simulink library "AEMS_Standard_Library"  (R2016b)
settings: Solver=ode45  StartTime=0.0  StopTime=10.0  RelTol=1e-3
undefined symbols (not defined in the file or in its folder): BkPY, carto, Cbx_extegr, Cbx_lpegrsys, Cbx_portegr, Cnx_bnk_nr_conf, Cnx_cyl_nr_conf, ConfigManagement, configuration_management, Cxx_dcm_io_tmr_end_xxxx, Cxx_dcm_rt_tmr_end, Cxx_DID_xxxx_IO_max, Cxx_DID_xxxx_IO_min, Cxx_egrhsofs, Cxx_vmaniegi, DEM_DEBOUNCE_FREEZE, DEM_DTR_CTL_INVISIBLE, DEM_DTR_CTL_NORMAL, Dem_DtrId2_XXX, Dem_DtrId3_XXX, Dem_DtrId4_XXX, Dem_DtrId5_XXX, Dem_DtrId6_XXX, Dem_DtrId7_XXX, Dem_DtrId8_XXX, Dem_DtrId9_XXX, Dem_DtrId_XXX, Dem_EnableConditionId2_XXX, Dem_EnableConditionId3_XXX, Dem_EnableConditionId4_XXX, Dem_EnableConditionId5_XXX, Dem_EnableConditionId6_XXX, Dem_EnableConditionId7_XXX, Dem_EnableConditionId8_XXX, Dem_EnableConditionId_XXX, Dem_EventId, Dem_EventId2_XXX, Dem_EventId3_XXX, Dem_EventId4_XXX, Dem_EventId5_XXX, Dem_EventId6_XXX, Dem_EventId7_XXX, Dem_EventId8_XXX, Dem_EventId9_XXX, Dem_EventId_Device_Faulttype, Dem_EventId_XXX, DEM_IUMPR_GENERAL_DENOMINATOR, DEM_OPCYC_IGNITION, Dem_RatioId2_XXX, Dem_RatioId3_XXX, Dem_RatioId4_XXX, Dem_RatioId5_XXX, Dem_RatioId6_XXX, Dem_RatioId7_XXX, Dem_RatioId8_XXX, Dem_RatioId_XXX, Dem_StorageConditionId2_XXX, Dem_StorageConditionId3_XXX, Dem_StorageConditionId4_XXX, Dem_StorageConditionId5_XXX ... (+65)
libraries: AEMS_Standard_Library x477, simulink x2
(part 19 of 39)

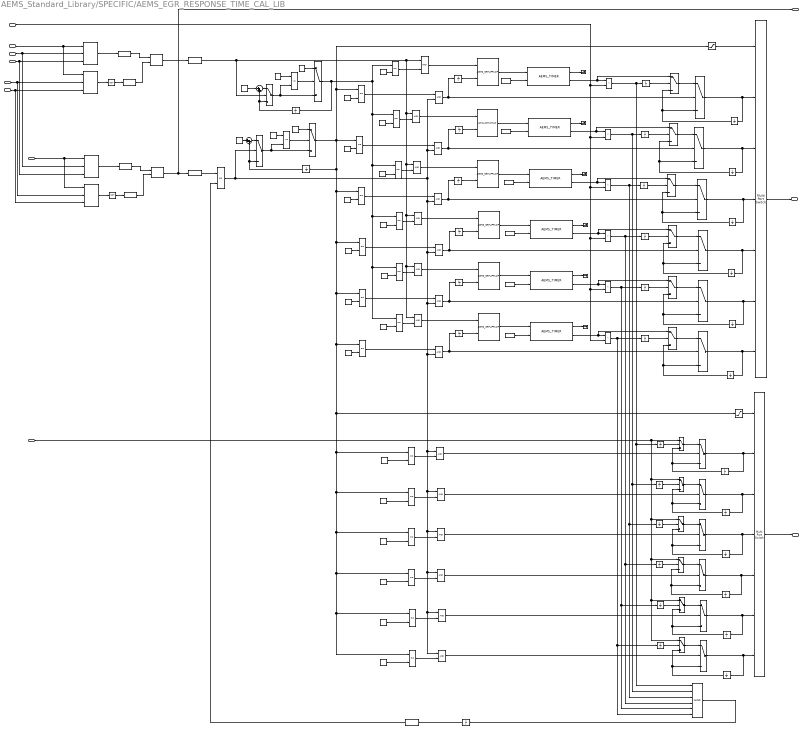
== system AEMS_Standard_Library/SPECIFIC/AEMS_EGR_RESPONSE_TIME_CAL_LIB ==
  timeup_time : Inport  PortDimensions=1
      settings: AttributesFormatString=<tsample=%<SampleTime>>
  etdamsf : Inport  Port=2  PortDimensions=1
      settings: AttributesFormatString=<tsample=%<SampleTime>>
  goal_trig_parameter : Inport  Port=3  PortDimensions=1
      settings: AttributesFormatString=<tsample=%<SampleTime>>
  start_trig_parameter : Inport  Port=4  PortDimensions=1
      settings: AttributesFormatString=<tsample=%<SampleTime>>
  on_thrs : Inport  Port=5  PortDimensions=1
      settings: AttributesFormatString=<tsample=%<SampleTime>>
  off_thrs : Inport  Port=6  PortDimensions=1
      settings: AttributesFormatString=<tsample=%<SampleTime>>
  on_hysw : Inport  Port=7  PortDimensions=1
      settings: AttributesFormatString=<tsample=%<SampleTime>>
  off_hysw : Inport  Port=8  PortDimensions=1
      settings: AttributesFormatString=<tsample=%<SampleTime>>
  AEMS_EDGE_EITHER1 : AEMS_Standard_Library/EDGE/AEMS_EDGE_EITHER  Tag=[LIB]  init=false
      settings: AttributesFormatString=|
      | %<MaskType>
      | Initial Value : %<init>
  AEMS_EDGE_EITHER2 : AEMS_Standard_Library/EDGE/AEMS_EDGE_EITHER  Tag=[LIB]  init=false
      settings: AttributesFormatString=|
      | %<MaskType>
      | Initial Value : %<init>
  AEMS_EDGE_RISING{,1..4} (5 alike) : AEMS_Standard_Library/EDGE/AEMS_EDGE_RISING  Tag=[LIB]  init=false
      settings: AttributesFormatString=|
      | %<MaskType>
      | Initial Value : %<init>
  AEMS_HYST_DELTARIGHT1 : AEMS_Standard_Library/HYSTERESIS/AEMS_HYST_DELTARIGHT  Tag=[LIB]
      settings: AttributesFormatString=%<MaskType>
  AEMS_HYST_DELTARIGHT2 : AEMS_Standard_Library/HYSTERESIS/AEMS_HYST_DELTARIGHT  Tag=[LIB]
      settings: AttributesFormatString=%<MaskType>
  AEMS_HYST_LEFTDELTA1 : AEMS_Standard_Library/HYSTERESIS/AEMS_HYST_LEFTDELTA  Tag=[LIB]
      settings: AttributesFormatString=%<MaskType>
  AEMS_HYST_LEFTDELTA2 : AEMS_Standard_Library/HYSTERESIS/AEMS_HYST_LEFTDELTA  Tag=[LIB]
      settings: AttributesFormatString=%<MaskType>
  AEMS_SRFLIPFLOP{,1..7} (8 alike) : AEMS_Standard_Library/FLAG/AEMS_SRFLIPFLOP  Tag=[LIB]  init=false
      settings: AttributesFormatString=%<MaskType>\nInitial condition (state of Q): = %<init>
  AEMS_TIMER{,1..5} (6 alike) : AEMS_Standard_Library/TIMER/AEMS_TIMER  Tag=[LIB]  sample_time=0.01
      settings: AttributesFormatString=%<MaskType>
  Constant10 : Constant  Value=6  OutDataTypeStr=uint8
  Constant11 : Constant  Value=6  OutDataTypeStr=uint8
  Constant12 : Constant  Value=4  OutDataTypeStr=uint8
  Constant13 : Constant  Value=5  OutDataTypeStr=uint8
  Constant14 : Constant  Value=6  OutDataTypeStr=uint8
  Constant{3,6,9,16..18} (6 alike) : Constant  OutDataTypeStr=single
  Constant{19,21..22,25,29,32..33} (7 alike) : Constant  OutDataTypeStr=uint8
  Constant20 : Constant  Value=7  OutDataTypeStr=uint8
  Constant23 : Constant  Value=2  OutDataTypeStr=uint8
  Constant24 : Constant  Value=3  OutDataTypeStr=uint8
  Constant26 : Constant  Value=2  OutDataTypeStr=uint8
  Constant27 : Constant  Value=3  OutDataTypeStr=uint8
  Constant28 : Constant  Value=7  OutDataTypeStr=uint8
  Constant30 : Constant  Value=3  OutDataTypeStr=uint8
  Constant31 : Constant  Value=2  OutDataTypeStr=uint8
  Constant4 : Constant  Value=4  OutDataTypeStr=uint8
  Constant5 : Constant  Value=4  OutDataTypeStr=uint8
  Constant7 : Constant  Value=5  OutDataTypeStr=uint8
  Constant8 : Constant  Value=5  OutDataTypeStr=uint8
  Logical Operator{1,4..11,13,17,19,24..29} (18 alike) : Logic  OutDataTypeStr=boolean
  Logical Operator12 : Logic  Operator=NOT  OutDataTypeStr=boolean
  Logical Operator18 : Logic  Operator=NAND  Inputs=6  OutDataTypeStr=boolean
  Logical Operator2 : Logic  Operator=OR  OutDataTypeStr=boolean
  Logical Operator3 : Logic  Operator=NOT  OutDataTypeStr=boolean
  Multiport Switch : MultiPortSwitch  Inputs=6  SaturateOnIntegerOverflow=on  InputSameDT=on
  Multiport Switch1 : MultiPortSwitch  Inputs=6  SaturateOnIntegerOverflow=on  InputSameDT=on
  Relational Operator{2,5..6,8,10..14,20,22..23,25..26,28..31} (18 alike) : RelationalOperator  Operator===  OutDataTypeStr=boolean  RndMeth=Nearest  InputSameDT=on
  Relational Operator{16,18..19,21,24,27} (6 alike) : RelationalOperator  Operator=<  OutDataTypeStr=boolean  RndMeth=Nearest  InputSameDT=on
  Relational Operator7 : RelationalOperator  Operator=<=  OutDataTypeStr=boolean  RndMeth=Nearest  InputSameDT=on
  Relational Operator9 : RelationalOperator  Operator=<=  OutDataTypeStr=boolean  RndMeth=Nearest  InputSameDT=on
  Saturation : Saturate  UpperLimit=6  LowerLimit=1
      settings: AttributesFormatString=<limits=%<UpperLimit>/%<LowerLimit>>
  Saturation1 : Saturate  UpperLimit=6  LowerLimit=1
      settings: AttributesFormatString=<limits=%<UpperLimit>/%<LowerLimit>>
  Sum1 : Sum  Inputs=|++  SaturateOnIntegerOverflow=on
  Sum2 : Sum  Inputs=|++  SaturateOnIntegerOverflow=on
  Switch{,1..10,12..13,15..17,20..31} (28 alike) : Switch  Threshold=0.5  SaturateOnIntegerOverflow=on  InputSameDT=on
      Switch settings: AttributesFormatString=<Threshold=%<Threshold>>
      Switch1 settings: AttributesFormatString=<threshold=%<threshold>>
      Switch10 settings: AttributesFormatString=<threshold=%<threshold>>
      Switch12 settings: AttributesFormatString=<threshold=%<threshold>>
      Switch13 settings: AttributesFormatString=<threshold=%<threshold>>
      Switch15 settings: AttributesFormatString=<Threshold=%<Threshold>>
      Switch16 settings: AttributesFormatString=<Threshold=%<Threshold>>
      Switch17 settings: AttributesFormatString=<Threshold=%<Threshold>>
      Switch2 settings: AttributesFormatString=<Threshold=%<Threshold>>
      Switch20 settings: AttributesFormatString=<Threshold=%<Threshold>>
      Switch21 settings: AttributesFormatString=<Threshold=%<Threshold>>
      Switch22 settings: AttributesFormatString=<Threshold=%<Threshold>>
      Switch23 settings: AttributesFormatString=<Threshold=%<Threshold>>
      Switch24 settings: AttributesFormatString=<Threshold=%<Threshold>>
      Switch25 settings: AttributesFormatString=<Threshold=%<Threshold>>
      Switch26 settings: AttributesFormatString=<threshold=%<threshold>>
      Switch27 settings: AttributesFormatString=<threshold=%<threshold>>
      Switch28 settings: AttributesFormatString=<threshold=%<threshold>>
      Switch29 settings: AttributesFormatString=<threshold=%<threshold>>
      Switch3 settings: AttributesFormatString=<Threshold=%<Threshold>>
      Switch30 settings: AttributesFormatString=<threshold=%<threshold>>
      Switch31 settings: AttributesFormatString=<threshold=%<threshold>>
      Switch4 settings: AttributesFormatString=<threshold=%<threshold>>
      Switch5 settings: AttributesFormatString=<threshold=%<threshold>>
      Switch6 settings: AttributesFormatString=<threshold=%<threshold>>
      Switch7 settings: AttributesFormatString=<threshold=%<threshold>>
      Switch8 settings: AttributesFormatString=<threshold=%<threshold>>
      Switch9 settings: AttributesFormatString=<threshold=%<threshold>>
  Terminator{,1..5} (6 alike) : Terminator
  Unit Delay{,1,3,7..14,16..23,25..38} (33 alike) : UnitDelay  SampleTime=-1
      settings: AttributesFormatString=<initial=%<X0>>
  fegrqinc : Outport  PortDimensions=1
  egrqpassdt : Outport  Port=2  PortDimensions=1
  etdamsf_store : Outport  Port=3  PortDimensions=1
  wires:
  Unit Delay14/1 -> Sum1/2, Switch12/3  "count_pudt"
  Unit Delay1/1 -> Sum2/2, Switch1/3  "count1_pudt"
  AEMS_SRFLIPFLOP6/1 -> fegrqinc/1, AEMS_EDGE_EITHER2/1  "fegrqinc"
  AEMS_EDGE_RISING4/1 -> AEMS_SRFLIPFLOP6/2
  AEMS_EDGE_RISING3/1 -> AEMS_SRFLIPFLOP6/1
  Logical Operator12/1 -> AEMS_EDGE_RISING4/1  "flag"
  AEMS_HYST_LEFTDELTA2/1 -> Logical Operator12/1  "egrq0_off"
  AEMS_HYST_DELTARIGHT2/1 -> AEMS_EDGE_RISING3/1  "egrq0_on"
  goal_trig_parameter/1 -> AEMS_HYST_LEFTDELTA2/1, AEMS_HYST_DELTARIGHT2/1  "goal_trig_parameter"
  off_thrs/1 -> AEMS_HYST_LEFTDELTA2/2, AEMS_HYST_LEFTDELTA1/2  "off_thrs"
  AEMS_EDGE_RISING2/1 -> AEMS_SRFLIPFLOP3/2
  AEMS_EDGE_RISING/1 -> AEMS_SRFLIPFLOP3/1
  Logical Operator3/1 -> AEMS_EDGE_RISING2/1  "flag"
  AEMS_HYST_LEFTDELTA1/1 -> Logical Operator3/1  "egrq0_off"
  off_hysw/1 -> AEMS_HYST_LEFTDELTA2/3, AEMS_HYST_LEFTDELTA1/3  "off_hysw"
  AEMS_HYST_DELTARIGHT1/1 -> AEMS_EDGE_RISING/1  "egrq0_on"
  on_hysw/1 -> AEMS_HYST_DELTARIGHT2/3, AEMS_HYST_DELTARIGHT1/3  "on_hysw"
  on_thrs/1 -> AEMS_HYST_DELTARIGHT2/2, AEMS_HYST_DELTARIGHT1/2  "on_thrs"
  start_trig_parameter/1 -> AEMS_HYST_DELTARIGHT1/1, AEMS_HYST_LEFTDELTA1/1  "start_trig_parameter"
  AEMS_EDGE_RISING1/1 -> Logical Operator2/2
  Switch/1 -> Unit Delay/1, Multiport Switch1/2  "holdtime1"
  AEMS_TIMER/1 -> Terminator/1
  Constant18/1 -> AEMS_TIMER/2  "target_time"
  Switch12/1 -> Relational Operator9/2, Switch13/3  "add"
  Constant20/1 -> Relational Operator9/1
  Constant21/1 -> Switch13/1
  Relational Operator9/1 -> Switch13/2
  Switch13/1 -> Relational Operator10/1, Relational Operator11/1, Relational Operator20/1, Relational Operator23/1, Relational Operator26/1, Relational Operator14/1, Unit Delay14/1  "count"
  Relational Operator14/1 -> Logical Operator4/2
  Constant22/1 -> Relational Operator14/2
  Constant23/1 -> Relational Operator10/2
  Relational Operator10/1 -> Logical Operator6/2
  Constant24/1 -> Relational Operator11/2
  Relational Operator11/1 -> Logical Operator7/2
  Constant19/1 -> Sum1/1
  Sum1/1 -> Switch12/1
  Switch2/1 -> Multiport Switch1/3, Unit Delay7/1  "holdtime2"
  AEMS_TIMER1/1 -> Terminator1/1
  Constant16/1 -> AEMS_TIMER1/2  "target_time"
  Switch3/1 -> Unit Delay8/1, Multiport Switch1/4  "holdtime3"
  AEMS_TIMER2/1 -> Terminator2/1
  Constant17/1 -> AEMS_TIMER2/2  "target_time"
  Unit Delay9/1 -> Switch9/3, Switch4/3  "hold2_z"
  Switch4/1 -> Unit Delay9/1, Multiport Switch/3  "hold2"
  Constant26/1 -> Relational Operator2/2
  Unit Delay11/1 -> Switch10/3, Switch6/3  "hold3_z"
  Switch6/1 -> Unit Delay11/1, Multiport Switch/4  "hold3"
  Constant27/1 -> Relational Operator6/2
  Switch5/1 -> Unit Delay10/1, Multiport Switch/2  "hold1"
  Unit Delay10/1 -> Switch5/3, Switch8/3  "hod1_z"
  Saturation/1 -> Multiport Switch/1
  Constant25/1 -> Relational Operator5/2
  Saturation1/1 -> Multiport Switch1/1
  Multiport Switch/1 -> etdamsf_store/1  "etdamsf_store"
  AEMS_SRFLIPFLOP/1 -> AEMS_TIMER/1  "start_flag"
  Logical Operator4/1 -> AEMS_SRFLIPFLOP/1  "set"
  Logical Operator8/1 -> Unit Delay13/1, Switch/2  "fhold1"
  AEMS_SRFLIPFLOP1/1 -> AEMS_TIMER1/1  "start_flag"
  Logical Operator6/1 -> AEMS_SRFLIPFLOP1/1  "set"
  AEMS_SRFLIPFLOP2/1 -> AEMS_TIMER2/1  "start_flag"
  Logical Operator7/1 -> AEMS_SRFLIPFLOP2/1  "set"
  Logical Operator5/1 -> Unit Delay12/1, Switch2/2  "fhold2"
  Logical Operator1/1 -> Unit Delay3/1, Switch3/2  "fhold3"
  Switch1/1 -> Switch7/3, Relational Operator7/2  "add1"
  Constant28/1 -> Relational Operator7/1
  Constant29/1 -> Switch7/1
  Relational Operator7/1 -> Switch7/2
  Sum2/1 -> Switch1/1
  Constant30/1 -> Relational Operator8/2
  Constant31/1 -> Relational Operator12/2
  Constant32/1 -> Relational Operator13/2
  Relational Operator8/1 -> Logical Operator1/1  "store_clear3"
  Relational Operator13/1 -> Logical Operator8/1  "store_clear1"
  Relational Operator12/1 -> Logical Operator5/1  "store_clear2"
  Relational Operator5/1 -> Logical Operator9/2
  Logical Operator9/1 -> Switch5/2
  Relational Operator2/1 -> Logical Operator10/2
  Logical Operator10/1 -> Switch4/2
  Relational Operator6/1 -> Logical Operator11/2
  Logical Operator11/1 -> Switch6/2
  Unit Delay3/1 -> AEMS_SRFLIPFLOP2/2  "clear"
  Unit Delay12/1 -> AEMS_SRFLIPFLOP1/2  "clear"
  Unit Delay13/1 -> AEMS_SRFLIPFLOP/2  "clear"
  Unit Delay/1 -> Switch/3, Switch16/3  "holdtime1_z"
  Unit Delay8/1 -> Switch3/3, Switch17/3  "holdtime3_z"
  Multiport Switch1/1 -> egrqpassdt/1  "egrqpassdt"
  AEMS_TIMER1/2 -> Relational Operator16/1, Switch15/1
  Relational Operator16/1 -> Unit Delay17/1, Unit Delay22/1, Logical Operator18/2  "timeok2"
  Unit Delay7/1 -> Switch15/3, Switch2/3  "holdtime2_z"
  Switch15/1 -> Switch2/1
  Constant33/1 -> Sum2/1
  Logical Operator18/1 -> Unit Delay18/1  "ftimeover"
  Logical Operator2/1 -> Switch1/2, Logical Operator8/2, Logical Operator5/2, Logical Operator1/2, Logical Operator13/2, Logical Operator19/2, Logical Operator25/2, Logical Operator9/1, Logical Operator11/1, Logical Operator27/1, Logical Operator28/1, Logical Operator29/1, Logical Operator10/1  "time_stop"
  Unit Delay18/1 -> AEMS_EDGE_RISING1/1  "flag"
  Relational Operator18/1 -> Unit Delay23/1, Logical Operator18/3, Unit Delay20/1  "timeok3"
  Switch17/1 -> Switch3/1
  AEMS_TIMER2/2 -> Relational Operator18/1, Switch17/1
  AEMS_TIMER/2 -> Switch16/1, Relational Operator19/1
  Switch16/1 -> Switch/1
  Relational Operator19/1 -> Unit Delay21/1, Logical Operator18/1, Unit Delay19/1  "timeok1"
  timeup_time/1 -> Relational Operator16/2, Relational Operator18/2, Relational Operator21/2, Relational Operator24/2, Relational Operator27/2, Relational Operator19/2  "timeup_time"
  Switch8/1 -> Switch5/1
  Switch9/1 -> Switch4/1
  Switch10/1 -> Switch6/1
  etdamsf/1 -> Switch8/1, Switch9/1, Switch10/1, Switch26/1, Switch28/1, Switch30/1  "etdamsf"
  AEMS_SRFLIPFLOP3/1 -> AEMS_EDGE_EITHER1/1  "flag"
  AEMS_EDGE_EITHER1/1 -> Switch12/2, Logical Operator4/1, Logical Operator6/1, Logical Operator7/1, Logical Operator17/1, Logical Operator24/1, Logical Operator26/1  "set_trig"
  AEMS_EDGE_EITHER2/1 -> Logical Operator2/1
  Unit Delay17/1 -> Switch15/2
  Unit Delay19/1 -> Switch16/2
  Unit Delay20/1 -> Switch17/2
  Unit Delay21/1 -> Switch8/2
  Unit Delay22/1 -> Switch9/2
  Unit Delay23/1 -> Switch10/2
  Switch7/1 -> Relational Operator12/1, Unit Delay1/1, Relational Operator8/1, Relational Operator22/1, Relational Operator25/1, Relational Operator28/1, Relational Operator5/1, Relational Operator2/1, Relational Operator6/1, Relational Operator29/1, Relational Operator30/1, Relational Operator31/1, Saturation/1, Relational Operator13/1, Saturation1/1  "count1"
  Relational Operator20/1 -> Logical Operator17/2
  Switch21/1 -> Unit Delay26/1, Multiport Switch1/5  "holdtime4"
  AEMS_TIMER3/1 -> Terminator3/1
  Constant3/1 -> AEMS_TIMER3/2  "target_time"
  AEMS_SRFLIPFLOP4/1 -> AEMS_TIMER3/1  "start_flag"
  Logical Operator17/1 -> AEMS_SRFLIPFLOP4/1  "set"
  Logical Operator13/1 -> Unit Delay25/1, Switch21/2  "fhold4"
  Constant5/1 -> Relational Operator22/2
  Relational Operator22/1 -> Logical Operator13/1  "store_clear4"
  Unit Delay25/1 -> AEMS_SRFLIPFLOP4/2  "clear"
  Unit Delay26/1 -> Switch21/3, Switch20/3  "holdtime4_z"
  Switch20/1 -> Switch21/1
  AEMS_TIMER3/2 -> Relational Operator21/1, Switch20/1
  Unit Delay16/1 -> Switch20/2
  Relational Operator23/1 -> Logical Operator24/2
  AEMS_TIMER4/1 -> Terminator4/1
  Constant6/1 -> AEMS_TIMER4/2  "target_time"
  AEMS_SRFLIPFLOP5/1 -> AEMS_TIMER4/1  "start_flag"
  Logical Operator24/1 -> AEMS_SRFLIPFLOP5/1  "set"
  Logical Operator19/1 -> Unit Delay28/1, Switch23/2  "fhold5"
  Constant8/1 -> Relational Operator25/2
  Relational Operator25/1 -> Logical Operator19/1  "store_clear5"
  Unit Delay28/1 -> AEMS_SRFLIPFLOP5/2  "clear"
  Unit Delay29/1 -> Switch23/3, Switch22/3  "holdtime5_z"
  Switch22/1 -> Switch23/1
  AEMS_TIMER4/2 -> Relational Operator24/1, Switch22/1
  Unit Delay27/1 -> Switch22/2
  Relational Operator26/1 -> Logical Operator26/2
  AEMS_TIMER5/1 -> Terminator5/1
  Constant9/1 -> AEMS_TIMER5/2  "target_time"
  AEMS_SRFLIPFLOP7/1 -> AEMS_TIMER5/1  "start_flag"
  Logical Operator26/1 -> AEMS_SRFLIPFLOP7/1  "set"
  Logical Operator25/1 -> Unit Delay31/1, Switch25/2  "fhold6"
  Constant11/1 -> Relational Operator28/2
  Relational Operator28/1 -> Logical Operator25/1  "store_clear6"
  Unit Delay31/1 -> AEMS_SRFLIPFLOP7/2  "clear"
  Unit Delay32/1 -> Switch25/3, Switch24/3  "holdtime6_z"
  Switch24/1 -> Switch25/1
  AEMS_TIMER5/2 -> Relational Operator27/1, Switch24/1
  Unit Delay30/1 -> Switch24/2
  Constant4/1 -> Relational Operator20/2
  Constant7/1 -> Relational Operator23/2
  Constant10/1 -> Relational Operator26/2
  Switch25/1 -> Multiport Switch1/7, Unit Delay32/1  "holdtime6"
  Switch23/1 -> Multiport Switch1/6, Unit Delay29/1  "holdtime5"
  Unit Delay33/1 -> Switch26/3, Switch27/3  "hold4_z"
  Switch27/1 -> Unit Delay33/1, Multiport Switch/5  "hold4"
  Constant12/1 -> Relational Operator29/2
  Relational Operator29/1 -> Logical Operator27/2
  Logical Operator27/1 -> Switch27/2
  Switch26/1 -> Switch27/1
  Unit Delay34/1 -> Switch26/2
  Unit Delay35/1 -> Switch28/3, Switch29/3  "hold5_z"
  Constant13/1 -> Relational Operator30/2
  Relational Operator30/1 -> Logical Operator28/2
  Logical Operator28/1 -> Switch29/2
  Switch28/1 -> Switch29/1
  Unit Delay36/1 -> Switch28/2
  Unit Delay37/1 -> Switch30/3, Switch31/3  "hold6_z"
  Constant14/1 -> Relational Operator31/2
  Relational Operator31/1 -> Logical Operator29/2
  Logical Operator29/1 -> Switch31/2
  Switch30/1 -> Switch31/1
  Unit Delay38/1 -> Switch30/2
  Switch29/1 -> Multiport Switch/6, Unit Delay35/1  "hold5"
  Switch31/1 -> Multiport Switch/7, Unit Delay37/1  "hold6"
  Relational Operator27/1 -> Unit Delay30/1, Unit Delay38/1, Logical Operator18/6  "timeok6"
  Relational Operator24/1 -> Unit Delay27/1, Unit Delay36/1, Logical Operator18/5  "timeok5"
  Relational Operator21/1 -> Unit Delay34/1, Logical Operator18/4, Unit Delay16/1  "timeok4"

== system AEMS_Standard_Library/SPECIFIC/AEMS_INTERP_WITH_BREAKPOINT ==
  map1 : Inport  Interpolate=off
  map2 : Inport  Port=2  Interpolate=off
  rax1 : Inport  Port=3  Interpolate=off
  rax2 : Inport  Port=4  Interpolate=off
  value : Inport  Port=5  Interpolate=off
  tolerance : Inport  Port=6  Interpolate=off
  AEMS_UL_INTERP : AEMS_Standard_Library/SPECIFIC/AEMS_UL_INTERP  Tag=[LIB]  Description=This library calculates interpolation for 2 inputs.
      settings: AttributesFormatString=%<MaskType>
  Constant : Constant  Value=0.00001  OutDataTypeStr=Inherit: Inherit via back propagation
  Divide : Product  Inputs=*/  OutDataTypeStr=Inherit: Inherit via back propagation
  MinMax1 : MinMax  Function=max  Inputs=2  SaturateOnIntegerOverflow=on  InputSameDT=on
  MinMax2 : MinMax  Function=max  Inputs=2  SaturateOnIntegerOverflow=on  InputSameDT=on
  Relational Operator : RelationalOperator  Operator=<=  OutDataTypeStr=boolean  RndMeth=Nearest  InputSameDT=on
  Sum : Sum  Inputs=+-  SaturateOnIntegerOverflow=on  InputSameDT=on
  Sum1 : Sum  Inputs=-+  SaturateOnIntegerOverflow=on  InputSameDT=on
  Switch{,1..3} (4 alike) : Switch  Criteria=u2 ~= 0  SaturateOnIntegerOverflow=on  InputSameDT=on
      settings: AttributesFormatString=Criteria=%<Criteria>
  output : Outport
  wires:
  Constant/1 -> MinMax2/2
  tolerance/1 -> MinMax2/1
  MinMax2/1 -> MinMax1/2
  AEMS_UL_INTERP/1 -> output/1
  value/1 -> Sum/1
  MinMax1/1 -> Divide/2
  Divide/1 -> AEMS_UL_INTERP/2
  Switch1/1 -> AEMS_UL_INTERP/1
  map2/1 -> Switch1/1, Switch3/3
  map1/1 -> Switch1/3, Switch3/1
  Relational Operator/1 -> Switch/2, Switch1/2, Switch2/2, Switch3/2
  rax1/1 -> Switch/1, Relational Operator/1, Switch2/3
  rax2/1 -> Relational Operator/2, Switch2/1, Switch/3
  Switch/1 -> Sum1/1, Sum/2
  Switch2/1 -> Sum1/2
  Sum1/1 -> MinMax1/1
  Sum/1 -> Divide/1
  Switch3/1 -> AEMS_UL_INTERP/3

== system AEMS_Standard_Library/SPECIFIC/AEMS_LOOKUP_LIBRARY ==
  ref_val : Inport
  tbl : Inport  Port=2
  brk_pt : Inport  Port=3
  len_tbl : Inport  Port=4
  Lookup_library : Stateflow chart
      settings: RTWSystemCode=Nonreusable function
  output_hi : Outport
  dlt1 : Outport  Port=2
  dlt2 : Outport  Port=3
  output_lo : Outport  Port=4
  wires:
  ref_val/1 -> Lookup_library/1(ref_val)
  tbl/1 -> Lookup_library/2(tbl)
  brk_pt/1 -> Lookup_library/3(brk_pt)
  len_tbl/1 -> Lookup_library/4(len_tbl)
  Lookup_library/1(output_hi) -> output_hi/1
  Lookup_library/2(dlt1) -> dlt1/1
  Lookup_library/3(dlt2) -> dlt2/1
  Lookup_library/4(output_lo) -> output_lo/1

== system AEMS_Standard_Library/SPECIFIC/AEMS_MULTIPORT_TIMESWITCH_CONFIG ==
  Duration : Inport
  Select_Input : Inport  Port=2
  Inputs : Inport  Port=3
  dT : Inport  Port=4
  AEMS_DIVISION_BY_ZERO : AEMS_Standard_Library/MATH/AEMS_DIVISION_BY_ZERO  Tag=[LIB]  Tolerence=1.1920929e-07
      settings: AttributesFormatString=%<MaskType>\nDenominator Tolerance = %<Tolerence>
  Constant2 : Constant  OutDataTypeStr=Inherit: Inherit via back propagation
  Get_input_and_input_old : Subsystem
  Saturation : Saturate  UpperLimit=LimitDimInputs  LowerLimit=1  RndMeth=Zero
      settings: AttributesFormatString=<limits=%<UpperLimit>/%<LowerLimit>>
  Subtract1 : Sum  Inputs=+-  OutDataTypeStr=Inherit: Inherit via back propagation  RndMeth=Zero  InputSameDT=on
  Subtract2 : Sum  Inputs=+-  OutDataTypeStr=Inherit: Inherit via back propagation  RndMeth=Zero  InputSameDT=on
  in_clc : Subsystem
  interpolation : Subsystem
  number_1_2 : Subsystem
  pulse_and_old : Subsystem
  slop_on : Subsystem
  transient_timer : Subsystem
  Output : Outport
  Slop_on : Outport  Port=2
  Ratio : Outport  Port=3
  wires:
  Inputs/1 -> Get_input_and_input_old/3(Inputs)
  transient_timer/1(Vxx_swi_trs) -> slop_on/1(Vxx_swi_trs), interpolation/4(Vxx_swi_trs)
  Get_input_and_input_old/2(Vxx_in_old) -> in_clc/4(Vxx_in_old)
  Get_input_and_input_old/1(Vxx_in) -> in_clc/3(Vxx_in)
  Saturation/1 -> Get_input_and_input_old/2(Select_Input), pulse_and_old/1(Select_Input)
  dT/1 -> transient_timer/2(dT)
  number_1_2/1(Vnx_swi_nr_stt) -> in_clc/1(Vnx_swi_nr_stt)
  pulse_and_old/2(Select_Input_old) -> Get_input_and_input_old/1(Select_Input_old)
  Duration/1 -> transient_timer/1(Duration)
  Select_Input/1 -> Saturation/1
  slop_on/1(Slop_on) -> Slop_on/1, interpolation/3(Slop_on), number_1_2/1(Slop_on)
  pulse_and_old/1(Vbx_sel_puls) -> transient_timer/3(Vbx_sel_puls), number_1_2/2(Vbx_sel_puls), in_clc/2(Vbx_sel_puls), slop_on/2(Vbx_sel_puls)
  Constant2/1 -> AEMS_DIVISION_BY_ZERO/3
  Subtract2/1 -> AEMS_DIVISION_BY_ZERO/1
  Subtract1/1 -> AEMS_DIVISION_BY_ZERO/2
  in_clc/2(Vxx_out_sel_old) -> Subtract2/2, Subtract1/2, interpolation/2(Vxx_out_sel_old)
  in_clc/1(Vxx_out_sel) -> Subtract2/1, interpolation/1(Vxx_out_sel)
  AEMS_DIVISION_BY_ZERO/1 -> Ratio/1
  interpolation/1(Output) -> Subtract1/1, Output/1

== system AEMS_Standard_Library/SPECIFIC/AEMS_OL_RATE_COUNTER ==
  frate_numerator : Inport
      settings: AttributesFormatString=<tsample=%<sampleTime>>
  frate_denominator : Inport  Port=2
      settings: AttributesFormatString=<tsample=%<sampleTime>>
  fdata_clear : Inport  Port=3
      settings: AttributesFormatString=<tsample=%<sampleTime>>
  OL_RATE_COUNTER : Stateflow chart  TreatAsAtomicUnit=on
  fcntend : Outport
  festrp : Outport  Port=2
  vrate_numerator : Outport  Port=3
  vrate_denominator : Outport  Port=4
  wires:
  frate_numerator/1 -> OL_RATE_COUNTER/1(frate_numerator)
  frate_denominator/1 -> OL_RATE_COUNTER/2(frate_denominator)
  fdata_clear/1 -> OL_RATE_COUNTER/3(fdata_clear)
  OL_RATE_COUNTER/1(fcntend) -> fcntend/1
  OL_RATE_COUNTER/4(vrate_denominator) -> vrate_denominator/1
  OL_RATE_COUNTER/3(vrate_numerator) -> vrate_numerator/1
  OL_RATE_COUNTER/2(festrp) -> festrp/1

== system AEMS_Standard_Library/SPECIFIC/AEMS_OL_RATE_COUNTER_B ==
  frate_numerator : Inport
  frate_denominator : Inport  Port=2
  fdata_clear : Inport  Port=3
  OL_RATE_COUNTER_B : Stateflow chart  TreatAsAtomicUnit=on
  fcntend : Outport
  festrp : Outport  Port=2
  vrate_numerator : Outport  Port=3
  vrate_denominator : Outport  Port=4
  wires:
  OL_RATE_COUNTER_B/2(festrp) -> festrp/1
  OL_RATE_COUNTER_B/4(vrate_denominator) -> vrate_denominator/1
  OL_RATE_COUNTER_B/3(vrate_numerator) -> vrate_numerator/1
  OL_RATE_COUNTER_B/1(fcntend) -> fcntend/1
  fdata_clear/1 -> OL_RATE_COUNTER_B/3(fdata_clear)
  frate_numerator/1 -> OL_RATE_COUNTER_B/1(frate_numerator)
  frate_denominator/1 -> OL_RATE_COUNTER_B/2(frate_denominator)

== system AEMS_Standard_Library/SPECIFIC/AEMS_OL_SIMILAR_CONDITION_CHECK ==
  engine_rev : Inport
  similar_engine_rev : Inport  Port=2
  load_value : Inport  Port=3
  similar_load_value : Inport  Port=4
  coolant_temp : Inport  Port=5
  similar_coolant_temp : Inport  Port=6
  Add1 : Sum  Inputs=+-  SaturateOnIntegerOverflow=on  InputSameDT=on
  Add2 : Sum  SaturateOnIntegerOverflow=on  InputSameDT=on
  Constant_375rpm : Constant  Value=375  OutDataTypeStr=Inherit: Inherit via back propagation
  Constant_70degC : Constant  Value=70  OutDataTypeStr=Inherit: Inherit via back propagation
  Gain_0.8 : Gain  Gain=0.8  SaturateOnIntegerOverflow=on  ParamDataTypeStr=Inherit: Same as input
  Gain_1.2 : Gain  Gain=1.2  SaturateOnIntegerOverflow=on  ParamDataTypeStr=Inherit: Same as input
  LogicalOperator1 : Logic  Operator=XOR  OutDataTypeStr=boolean
  LogicalOperator2 : Logic  Inputs=5  OutDataTypeStr=boolean
  RelationalOperator1 : RelationalOperator  OutDataTypeStr=boolean  RndMeth=Nearest  InputSameDT=on
  RelationalOperator2 : RelationalOperator  Operator=>  OutDataTypeStr=boolean  RndMeth=Nearest  InputSameDT=on
  RelationalOperator3 : RelationalOperator  OutDataTypeStr=boolean  RndMeth=Nearest  InputSameDT=on
  RelationalOperator4 : RelationalOperator  Operator=>  OutDataTypeStr=boolean  RndMeth=Nearest  InputSameDT=on
  RelationalOperator5 : RelationalOperator  OutDataTypeStr=boolean  RndMeth=Nearest  InputSameDT=on
  RelationalOperator6 : RelationalOperator  Operator=>  OutDataTypeStr=boolean  RndMeth=Nearest  InputSameDT=on
  similar_condition : Outport
  wires:
  Constant_70degC/1 -> RelationalOperator6/1, RelationalOperator5/2  "similar_coolant_temp_thres"
  Constant_375rpm/1 -> Add2/1, Add1/2  "similar_engine_rev_band"
  LogicalOperator2/1 -> similar_condition/1  "similar_condition"
  coolant_temp/1 -> RelationalOperator5/1  "coolant_temp"
  load_value/1 -> RelationalOperator4/2, RelationalOperator3/1  "load_value"
  engine_rev/1 -> RelationalOperator2/2, RelationalOperator1/1  "engine_rev"
  RelationalOperator4/1 -> LogicalOperator2/4
  RelationalOperator3/1 -> LogicalOperator2/3
  RelationalOperator2/1 -> LogicalOperator2/2
  RelationalOperator1/1 -> LogicalOperator2/1
  LogicalOperator1/1 -> LogicalOperator2/5
  RelationalOperator6/1 -> LogicalOperator1/2
  RelationalOperator5/1 -> LogicalOperator1/1
  similar_coolant_temp/1 -> RelationalOperator6/2  "similar_coolant_temp"
  similar_load_value/1 -> Gain_1.2/1, Gain_0.8/1  "similar_load_value"
  Gain_0.8/1 -> RelationalOperator3/2
  Gain_1.2/1 -> RelationalOperator4/1
  Add2/1 -> RelationalOperator2/1
  Add1/1 -> RelationalOperator1/2
  similar_engine_rev/1 -> Add2/2, Add1/1  "similar_engine_rev"

== system AEMS_Standard_Library/SPECIFIC/AEMS_OL_SIMILAR_CONDITION_SET ==
  erase : Inport
  mil : Inport  Port=2
  pending : Inport  Port=3
  rewrite : Inport  Port=4
  engine_rev : Inport  Port=5
  load_value : Inport  Port=6
  coolant_temp : Inport  Port=7
  OL_SIMILAR_CONDITION_SET : Stateflow chart
  similar_condition_set : Outport
  similar_engine_rev : Outport  Port=2
  similar_load_value : Outport  Port=3
  similar_coolant_temp : Outport  Port=4
  wires:
  erase/1 -> OL_SIMILAR_CONDITION_SET/1(erase)
  mil/1 -> OL_SIMILAR_CONDITION_SET/2(mil)
  pending/1 -> OL_SIMILAR_CONDITION_SET/3(pending)
  rewrite/1 -> OL_SIMILAR_CONDITION_SET/4(rewrite)
  engine_rev/1 -> OL_SIMILAR_CONDITION_SET/5(engine_rev)
  load_value/1 -> OL_SIMILAR_CONDITION_SET/6(load_value)
  coolant_temp/1 -> OL_SIMILAR_CONDITION_SET/7(coolant_temp)
  OL_SIMILAR_CONDITION_SET/1(similar_condition_set) -> similar_condition_set/1
  OL_SIMILAR_CONDITION_SET/2(similar_engine_rev) -> similar_engine_rev/1
  OL_SIMILAR_CONDITION_SET/3(similar_load_value) -> similar_load_value/1
  OL_SIMILAR_CONDITION_SET/4(similar_coolant_temp) -> similar_coolant_temp/1

== system AEMS_Standard_Library/SPECIFIC/AEMS_STATE_TRANSITION_SET_VALUE ==
  cont_transit_permit_times : Inport
  value : Inport  Port=2
  internal_ratio : Inport  Port=3
  value1 : Inport  Port=4
  internal_ratio2 : Inport  Port=5
  value2 : Inport  Port=6
  Constant1 : Constant  OutDataTypeStr=Inherit: Inherit via back propagation
  Constant3 : Constant  OutDataTypeStr=Inherit: Inherit via back propagation
  Constant5 : Constant  OutDataTypeStr=Inherit: Inherit via back propagation
  Product{1..4} (4 alike) : Product  OutDataTypeStr=Inherit: Inherit via back propagation  RndMeth=Zero
  Relational Operator3 : RelationalOperator  OutDataTypeStr=boolean  RndMeth=Nearest  InputSameDT=on
  Sum1 : Sum  Inputs=-+  SaturateOnIntegerOverflow=on  InputSameDT=on
  Sum2 : Sum  Inputs=-+  SaturateOnIntegerOverflow=on  InputSameDT=on
  Sum3 : Sum  SaturateOnIntegerOverflow=on  InputSameDT=on
  Sum4 : Sum  SaturateOnIntegerOverflow=on  InputSameDT=on
  Switch : Switch  Criteria=u2 ~= 0  SaturateOnIntegerOverflow=on  InputSameDT=on
      settings: AttributesFormatString=Criteria=%<Criteria>
  output : Outport
  wires:
  Relational Operator3/1 -> Switch/2
  cont_transit_permit_times/1 -> Relational Operator3/2  "cont_transit_permit_times"
  Constant3/1 -> Relational Operator3/1
  Sum4/1 -> Switch/3
  Switch/1 -> Product4/2
  value2/1 -> Product2/2  "value2"
  value1/1 -> Switch/1, Product1/1  "value1"
  Sum3/1 -> output/1  "output"
  value/1 -> Product3/1  "value"
  internal_ratio/1 -> Product3/2, Sum2/1  "internal_ratio"
  Constant5/1 -> Sum2/2
  Sum2/1 -> Product4/1
  Product3/1 -> Sum3/1
  Product4/1 -> Sum3/2
  Constant1/1 -> Sum1/2
  Sum1/1 -> Product2/1
  Product2/1 -> Sum4/2
  internal_ratio2/1 -> Sum1/1, Product1/2  "internal_ratio2"
  Product1/1 -> Sum4/1

== system AEMS_Standard_Library/SPECIFIC/AEMS_SUPPLIER_CALL_ANGL_DIF_SAME_BCH ==
  DataStoreRead : DataStoreRead  DataStoreName=Supplier_call_angl_dif_nxt_cyl
      settings: AttributesFormatString=<tsample=%<sampleTime>>
  Vxx_fms_angl_dif_nxt_cyl_lpos : Outport
  wires:
  DataStoreRead/1 -> Vxx_fms_angl_dif_nxt_cyl_lpos/1

== system AEMS_Standard_Library/SPECIFIC/AEMS_SUPPLIER_CALL_ESTI_TIME_INJ ==
  note: Splitnum
  note: Coding information: This block is to call Supplier call API.
      | Each block will be translated into code C by this way:
      | Output=Supplier call API Name(In,Splitnum);
      | Example for Supplier_Call_Esti_ti_main_post3, corresponding output variable is
      | Vxx_fms_esti_ti_wish_main_post3= Supplier_Call_Esti_ti_main_post3(In,3);
  In : Inport
  DataTypeConversion : DataTypeConversion
  Data_Store_Read : DataStoreRead  DataStoreName=Supplier_Call_Esti_ti_main_post2
      settings: AttributesFormatString=<tsample=%<sampleTime>>
  Splitnum : Constant  Value=2  OutDataTypeStr=uint8
  Terminator : Terminator
  Terminator1 : Terminator
  Vxx_fms_esti_ti_wish_main_post2 : Outport  InitialOutput=0
  wires:
  Splitnum/1 -> Terminator1/1
  In/1 -> Terminator/1
  Data_Store_Read/1 -> DataTypeConversion/1
  DataTypeConversion/1 -> Vxx_fms_esti_ti_wish_main_post2/1

== system AEMS_Standard_Library/SPECIFIC/AEMS_SUPPLIER_CALL_ESTI_TI_AFTR ==
  DataStoreRead : DataStoreRead  DataStoreName=Supplier_call_esti_ti_aftr
      settings: AttributesFormatString=<tsample=%<sampleTime>>
  Vxx_fms_esti_ti_aftr : Outport  InitialOutput=0
  wires:
  DataStoreRead/1 -> Vxx_fms_esti_ti_aftr/1

== system AEMS_Standard_Library/SPECIFIC/AEMS_SUPPLIER_CALL_ESTI_TI_LPOS ==
  DataStoreRead : DataStoreRead  DataStoreName=Supplier_call_esti_ti_lpos
      settings: AttributesFormatString=<tsample=%<sampleTime>>
  Vxx_fms_esti_ti_lpos : Outport  InitialOutput=0
  wires:
  DataStoreRead/1 -> Vxx_fms_esti_ti_lpos/1

== system AEMS_Standard_Library/SPECIFIC/AEMS_SUPPLIER_CALL_ESTI_TI_LPOS1_2SL ==
  DataStoreRead : DataStoreRead  DataStoreName=Supplier_call_esti_ti_lpos1_2sl
      settings: AttributesFormatString=<tsample=%<sampleTime>>
  Vxx_fms_esti_ti_lpos1_2sl : Outport  InitialOutput=0
  wires:
  DataStoreRead/1 -> Vxx_fms_esti_ti_lpos1_2sl/1

== system AEMS_Standard_Library/SPECIFIC/AEMS_SUPPLIER_CALL_ESTI_TI_LPOS1_3SL ==
  DataStoreRead : DataStoreRead  DataStoreName=Supplier_call_esti_ti_lpos1_3sl
      settings: AttributesFormatString=<tsample=%<sampleTime>>
  Vxx_fms_esti_ti_lpos1_3sl : Outport  InitialOutput=0
  wires:
  DataStoreRead/1 -> Vxx_fms_esti_ti_lpos1_3sl/1

== system AEMS_Standard_Library/SPECIFIC/AEMS_SUPPLIER_CALL_ESTI_TI_LPOS1_4SL ==
  DataStoreRead : DataStoreRead  DataStoreName=Supplier_call_esti_ti_lpos1_4sl
      settings: AttributesFormatString=<tsample=%<sampleTime>>
  Vxx_fms_esti_ti_lpos1_4sl : Outport  InitialOutput=0
  wires:
  DataStoreRead/1 -> Vxx_fms_esti_ti_lpos1_4sl/1

== system AEMS_Standard_Library/SPECIFIC/AEMS_SUPPLIER_CALL_ESTI_TI_LPOS2_2SL ==
  DataStoreRead : DataStoreRead  DataStoreName=Supplier_call_esti_ti_lpos2_2sl
      settings: AttributesFormatString=<tsample=%<sampleTime>>
  Vxx_fms_esti_ti_lpos2_2sl : Outport  InitialOutput=0
  wires:
  DataStoreRead/1 -> Vxx_fms_esti_ti_lpos2_2sl/1

== system AEMS_Standard_Library/SPECIFIC/AEMS_SUPPLIER_CALL_ESTI_TI_LPOS2_3SL ==
  DataStoreRead : DataStoreRead  DataStoreName=Supplier_call_esti_ti_lpos2_3sl
      settings: AttributesFormatString=<tsample=%<sampleTime>>
  Vxx_fms_esti_ti_lpos2_3sl : Outport  InitialOutput=0
  wires:
  DataStoreRead/1 -> Vxx_fms_esti_ti_lpos2_3sl/1

== system AEMS_Standard_Library/SPECIFIC/AEMS_SUPPLIER_CALL_ESTI_TI_LPOS2_4SL ==
  DataStoreRead : DataStoreRead  DataStoreName=Supplier_call_esti_ti_lpos2_4sl
      settings: AttributesFormatString=<tsample=%<sampleTime>>
  Vxx_fms_esti_ti_lpos2_4sl : Outport  InitialOutput=0
  wires:
  DataStoreRead/1 -> Vxx_fms_esti_ti_lpos2_4sl/1

== system AEMS_Standard_Library/SPECIFIC/AEMS_SUPPLIER_CALL_ESTI_TI_LPOS3_3SL ==
  DataStoreRead : DataStoreRead  DataStoreName=Supplier_call_esti_ti_lpos3_3sl
      settings: AttributesFormatString=<tsample=%<sampleTime>>
  Vxx_fms_esti_ti_lpos3_3sl : Outport  InitialOutput=0
  wires:
  DataStoreRead/1 -> Vxx_fms_esti_ti_lpos3_3sl/1

== system AEMS_Standard_Library/SPECIFIC/AEMS_SUPPLIER_CALL_ESTI_TI_LPOS3_4SL ==
  DataStoreRead : DataStoreRead  DataStoreName=Supplier_call_esti_ti_lpos3_4sl
      settings: AttributesFormatString=<tsample=%<sampleTime>>
  Vxx_fms_esti_ti_lpos3_4sl : Outport  InitialOutput=0
  wires:
  DataStoreRead/1 -> Vxx_fms_esti_ti_lpos3_4sl/1

== system AEMS_Standard_Library/SPECIFIC/AEMS_SUPPLIER_CALL_ESTI_TI_LPOS4_4SL ==
  DataStoreRead : DataStoreRead  DataStoreName=Supplier_call_esti_ti_lpos4_4sl
      settings: AttributesFormatString=<tsample=%<sampleTime>>
  Vxx_fms_esti_ti_lpos4_4sl : Outport  InitialOutput=0
  wires:
  DataStoreRead/1 -> Vxx_fms_esti_ti_lpos4_4sl/1

== system AEMS_Standard_Library/SPECIFIC/AEMS_SUPPLIER_CALL_ESTI_TI_MAIN ==
  DataStoreRead : DataStoreRead  DataStoreName=Supplier_call_esti_ti_main
      settings: AttributesFormatString=<tsample=%<sampleTime>>
  Vxx_fms_esti_ti_main : Outport  InitialOutput=0
  wires:
  DataStoreRead/1 -> Vxx_fms_esti_ti_main/1

== system AEMS_Standard_Library/SPECIFIC/AEMS_SUPPLIER_CALL_ESTI_TI_MAIN_AFTR ==
  DataStoreRead : DataStoreRead  DataStoreName=Supplier_call_esti_ti_main_aftr
      settings: AttributesFormatString=<tsample=%<sampleTime>>
  Vxx_fms_esti_ti_wish_main_aftr : Outport  InitialOutput=0
  wires:
  DataStoreRead/1 -> Vxx_fms_esti_ti_wish_main_aftr/1

== system AEMS_Standard_Library/SPECIFIC/AEMS_SUPPLIER_CALL_ESTI_TI_MAIN_POST ==
  DataStoreRead : DataStoreRead  DataStoreName=Supplier_call_esti_ti_main_post
      settings: AttributesFormatString=<tsample=%<sampleTime>>
  Vxx_fms_esti_ti_wish_main_post : Outport  InitialOutput=0
  wires:
  DataStoreRead/1 -> Vxx_fms_esti_ti_wish_main_post/1

== system AEMS_Standard_Library/SPECIFIC/AEMS_SUPPLIER_CALL_ESTI_TI_PINJ1 ==
  DataStoreRead : DataStoreRead  DataStoreName=Supplier_call_esti_ti_pinj1
      settings: AttributesFormatString=<tsample=%<sampleTime>>
  Vxx_fms_esti_ti_pinj1 : Outport
  wires:
  DataStoreRead/1 -> Vxx_fms_esti_ti_pinj1/1

== system AEMS_Standard_Library/SPECIFIC/AEMS_SUPPLIER_CALL_ESTI_TI_PINJ2 ==
  DataStoreRead : DataStoreRead  DataStoreName=Supplier_call_esti_ti_pinj2
      settings: AttributesFormatString=<tsample=%<sampleTime>>
  Vxx_fms_esti_ti_pinj2 : Outport
  wires:
  DataStoreRead/1 -> Vxx_fms_esti_ti_pinj2/1

== system AEMS_Standard_Library/SPECIFIC/AEMS_SUPPLIER_CALL_ESTI_TI_PINJ3 ==
  DataStoreRead : DataStoreRead  DataStoreName=Supplier_call_esti_ti_pinj3
      settings: AttributesFormatString=<tsample=%<sampleTime>>
  Vxx_fms_esti_ti_pinj3 : Outport
  wires:
  DataStoreRead/1 -> Vxx_fms_esti_ti_pinj3/1

== system AEMS_Standard_Library/SPECIFIC/AEMS_SUPPLIER_CALL_ESTI_TI_PINJ4 ==
  DataStoreRead : DataStoreRead  DataStoreName=Supplier_call_esti_ti_pinj4
      settings: AttributesFormatString=<tsample=%<sampleTime>>
  Vxx_fms_esti_ti_pinj4 : Outport
  wires:
  DataStoreRead/1 -> Vxx_fms_esti_ti_pinj4/1

== system AEMS_Standard_Library/SPECIFIC/AEMS_SUPPLIER_CALL_ESTI_TI_POST ==
  DataStoreRead : DataStoreRead  DataStoreName=Supplier_call_esti_ti_post
      settings: AttributesFormatString=<tsample=%<sampleTime>>
  Vxx_fms_esti_ti_post : Outport  InitialOutput=0
  wires:
  DataStoreRead/1 -> Vxx_fms_esti_ti_post/1

== system AEMS_Standard_Library/SPECIFIC/AEMS_SUPPLIER_CALL_FIM_MAX ==
  DataStoreRead : DataStoreRead  DataStoreName=Supplier_call_fim_max
      settings: AttributesFormatString=<tsample=%<sampleTime>>
  Vxx_fms_fim_tot_max : Outport  InitialOutput=0
  wires:
  DataStoreRead/1 -> Vxx_fms_fim_tot_max/1

== system AEMS_Standard_Library/SPECIFIC/AEMS_SUPPLIER_CALL_FIM_MIN_AFTR ==
  Data Store Read : DataStoreRead  DataStoreName=Supplier_call_fim_min
      settings: AttributesFormatString=<tsample=%<sampleTime>>
  Vxx_fms_fim_min_aftr : Outport  InitialOutput=0
  wires:
  Data Store Read/1 -> Vxx_fms_fim_min_aftr/1

== system AEMS_Standard_Library/SPECIFIC/AEMS_SUPPLIER_CALL_FIM_MIN_LPOS1 ==
  Data Store Read : DataStoreRead  DataStoreName=Supplier_call_fim_min
      settings: AttributesFormatString=<tsample=%<sampleTime>>
  Vxx_fms_fim_min_lpos1_1sl : Outport  InitialOutput=0
  wires:
  Data Store Read/1 -> Vxx_fms_fim_min_lpos1_1sl/1

== system AEMS_Standard_Library/SPECIFIC/AEMS_SUPPLIER_CALL_FIM_MIN_LPOS1_2SL ==
  Data Store Read : DataStoreRead  DataStoreName=Supplier_call_fim_min
      settings: AttributesFormatString=<tsample=%<sampleTime>>
  Vxx_fms_fim_min_lpos1_2sl : Outport  InitialOutput=0
  wires:
  Data Store Read/1 -> Vxx_fms_fim_min_lpos1_2sl/1

== system AEMS_Standard_Library/SPECIFIC/AEMS_SUPPLIER_CALL_FIM_MIN_LPOS1_3SL ==
  Data Store Read : DataStoreRead  DataStoreName=Supplier_call_fim_min
      settings: AttributesFormatString=<tsample=%<sampleTime>>
  Vxx_fms_fim_min_lpos1_3sl : Outport  InitialOutput=0
  wires:
  Data Store Read/1 -> Vxx_fms_fim_min_lpos1_3sl/1

== system AEMS_Standard_Library/SPECIFIC/AEMS_SUPPLIER_CALL_FIM_MIN_LPOS1_4SL ==
  Data Store Read : DataStoreRead  DataStoreName=Supplier_call_fim_min
      settings: AttributesFormatString=<tsample=%<sampleTime>>
  Vxx_fms_fim_min_lpos1_4sl : Outport  InitialOutput=0
  wires:
  Data Store Read/1 -> Vxx_fms_fim_min_lpos1_4sl/1

== system AEMS_Standard_Library/SPECIFIC/AEMS_SUPPLIER_CALL_FIM_MIN_LPOS2_2SL ==
  Data Store Read : DataStoreRead  DataStoreName=Supplier_call_fim_min
      settings: AttributesFormatString=<tsample=%<sampleTime>>
  Vxx_fms_fim_min_lpos2_2sl : Outport  InitialOutput=0
  wires:
  Data Store Read/1 -> Vxx_fms_fim_min_lpos2_2sl/1

== system AEMS_Standard_Library/SPECIFIC/AEMS_SUPPLIER_CALL_FIM_MIN_LPOS2_3SL ==
  Data Store Read : DataStoreRead  DataStoreName=Supplier_call_fim_min
      settings: AttributesFormatString=<tsample=%<sampleTime>>
  Vxx_fms_fim_min_lpos2_3sl : Outport  InitialOutput=0
  wires:
  Data Store Read/1 -> Vxx_fms_fim_min_lpos2_3sl/1

== system AEMS_Standard_Library/SPECIFIC/AEMS_SUPPLIER_CALL_FIM_MIN_LPOS2_4SL ==
  Data Store Read : DataStoreRead  DataStoreName=Supplier_call_fim_min
      settings: AttributesFormatString=<tsample=%<sampleTime>>
  Vxx_fms_fim_min_lpos2_4sl : Outport  InitialOutput=0
  wires:
  Data Store Read/1 -> Vxx_fms_fim_min_lpos2_4sl/1

== system AEMS_Standard_Library/SPECIFIC/AEMS_SUPPLIER_CALL_FIM_MIN_LPOS3_3SL ==
  Data Store Read : DataStoreRead  DataStoreName=Supplier_call_fim_min
      settings: AttributesFormatString=<tsample=%<sampleTime>>
  Vxx_fms_fim_min_lpos3_3sl : Outport  InitialOutput=0
  wires:
  Data Store Read/1 -> Vxx_fms_fim_min_lpos3_3sl/1

== system AEMS_Standard_Library/SPECIFIC/AEMS_SUPPLIER_CALL_FIM_MIN_LPOS3_4SL ==
  Data Store Read : DataStoreRead  DataStoreName=Supplier_call_fim_min
      settings: AttributesFormatString=<tsample=%<sampleTime>>
  Vxx_fms_fim_min_lpos3_4sl : Outport  InitialOutput=0
  wires:
  Data Store Read/1 -> Vxx_fms_fim_min_lpos3_4sl/1

== system AEMS_Standard_Library/SPECIFIC/AEMS_SUPPLIER_CALL_FIM_MIN_LPOS4_4SL ==
  Data Store Read : DataStoreRead  DataStoreName=Supplier_call_fim_min
      settings: AttributesFormatString=<tsample=%<sampleTime>>
  Vxx_fms_fim_min_lpos4_4sl : Outport  InitialOutput=0
  wires:
  Data Store Read/1 -> Vxx_fms_fim_min_lpos4_4sl/1

== system AEMS_Standard_Library/SPECIFIC/AEMS_SUPPLIER_CALL_FIM_MIN_MAIN ==
  Data Store Read : DataStoreRead  DataStoreName=Supplier_call_fim_min
      settings: AttributesFormatString=<tsample=%<sampleTime>>
  Vxx_fms_fim_min_main : Outport  InitialOutput=0
  wires:
  Data Store Read/1 -> Vxx_fms_fim_min_main/1

== system AEMS_Standard_Library/SPECIFIC/AEMS_SUPPLIER_CALL_FIM_MIN_PINJ1 ==
  Data Store Read : DataStoreRead  DataStoreName=Supplier_call_fim_min
      settings: AttributesFormatString=<tsample=%<sampleTime>>
  Vxx_fms_fim_min_pinj1 : Outport  InitialOutput=0
  wires:
  Data Store Read/1 -> Vxx_fms_fim_min_pinj1/1

== system AEMS_Standard_Library/SPECIFIC/AEMS_SUPPLIER_CALL_FIM_MIN_PINJ2 ==
  Data Store Read : DataStoreRead  DataStoreName=Supplier_call_fim_min
      settings: AttributesFormatString=<tsample=%<sampleTime>>
  Vxx_fms_fim_min_pinj2 : Outport  InitialOutput=0
  wires:
  Data Store Read/1 -> Vxx_fms_fim_min_pinj2/1

== system AEMS_Standard_Library/SPECIFIC/AEMS_SUPPLIER_CALL_FIM_MIN_PINJ3 ==
  Data Store Read : DataStoreRead  DataStoreName=Supplier_call_fim_min
      settings: AttributesFormatString=<tsample=%<sampleTime>>
  Vxx_fms_fim_min_pinj3 : Outport  InitialOutput=0
  wires:
  Data Store Read/1 -> Vxx_fms_fim_min_pinj3/1

== system AEMS_Standard_Library/SPECIFIC/AEMS_SUPPLIER_CALL_FIM_MIN_PINJ4 ==
  Data Store Read : DataStoreRead  DataStoreName=Supplier_call_fim_min
      settings: AttributesFormatString=<tsample=%<sampleTime>>
  Vxx_fms_fim_min_pinj4 : Outport  InitialOutput=0
  wires:
  Data Store Read/1 -> Vxx_fms_fim_min_pinj4/1

== system AEMS_Standard_Library/SPECIFIC/AEMS_SUPPLIER_CALL_FIM_MIN_POST ==
  Data Store Read : DataStoreRead  DataStoreName=Supplier_call_fim_min
      settings: AttributesFormatString=<tsample=%<sampleTime>>
  Vxx_fms_fim_min_post : Outport  InitialOutput=0
  wires:
  Data Store Read/1 -> Vxx_fms_fim_min_post/1

== system AEMS_Standard_Library/SPECIFIC/AEMS_SUPPLIER_CALL_FUEL_INJ_MIN ==
  note: Coding information: This block is to call Supplier call API.
      | Each block will be translated into code C by this way:
      | Output=Supplier call API Name(Splitnum);
      | Example for Supplier_Call_Fim_min_post1, corresponding output variable is
      | Vxx_fms_fim_min_post1= Supplier_Call_Fim_min_post1(1);
  note: Splitnum
  DataTypeConversion : DataTypeConversion
  Data_Store_Read : DataStoreRead  DataStoreName=Supplier_Call_Fim_min_post1
  Splitnum : Constant  Value=3  OutDataTypeStr=uint8
  Terminator2 : Terminator
  Vxx_fms_fim_min_post1_3sl : Outport  InitialOutput=0
  wires:
  Splitnum/1 -> Terminator2/1
  Data_Store_Read/1 -> DataTypeConversion/1
  DataTypeConversion/1 -> Vxx_fms_fim_min_post1_3sl/1

== system AEMS_Standard_Library/SPECIFIC/AEMS_SUPPLIER_CALL_ICLC_LEARNING ==
  ICLC_learning_SOI_1 : Inport
  ICLC_learning_MFF_raw : Inport  Port=2
  ICLC_learning_INJ_nr : Inport  Port=3
  Average_engine_speed : Inport  Port=4
  ICLC_disable_flag : Inport  Port=5
  ICLC_adaptation_reset_flag : Inport  Port=6
  DataStoreRead : DataStoreRead  DataStoreName=Supplier_call_ICLC_learning_request
  DataStoreRead1 : DataStoreRead  DataStoreName=Supplier_call_ICLC_learning_MFF_1
  Terminator{,1..5} (6 alike) : Terminator
  ICLC_learning_request : Outport  InitialOutput=0
  ICLC_learning_MFF_1 : Outport  Port=2  InitialOutput=0
  wires:
  DataStoreRead/1 -> ICLC_learning_request/1
  ICLC_learning_SOI_1/1 -> Terminator/1
  ICLC_learning_MFF_raw/1 -> Terminator1/1
  ICLC_learning_INJ_nr/1 -> Terminator2/1
  DataStoreRead1/1 -> ICLC_learning_MFF_1/1
  ICLC_adaptation_reset_flag/1 -> Terminator5/1
  ICLC_disable_flag/1 -> Terminator4/1
  Average_engine_speed/1 -> Terminator3/1

== system AEMS_Standard_Library/SPECIFIC/AEMS_SUPPLIER_CALL_MAX_NBR_INJ ==
  Data Store Read : DataStoreRead  DataStoreName=Supplier_call_nbr_inj_max
      settings: AttributesFormatString=<tsample=%<sampleTime>>
  Vxx_inj_cmd_max_nr : Outport  InitialOutput=0
  wires:
  Data Store Read/1 -> Vxx_inj_cmd_max_nr/1

== system AEMS_Standard_Library/SPECIFIC/AEMS_SUPPLIER_CALL_PHI_MAX_PINJ1 ==
  Data Store Read : DataStoreRead  DataStoreName=Supplier_Call_Phi_Max
      settings: AttributesFormatString=<tsample=%<sampleTime>>
  Vxx_fms_phi_max_pinj1 : Outport
  wires:
  Data Store Read/1 -> Vxx_fms_phi_max_pinj1/1

== system AEMS_Standard_Library/SPECIFIC/AEMS_SUPPLIER_CALL_PHI_MAX_PINJ2 ==
  Data Store Read : DataStoreRead  DataStoreName=Supplier_Call_Phi_Max
      settings: AttributesFormatString=<tsample=%<sampleTime>>
  Vxx_fms_phi_max_pinj2 : Outport
  wires:
  Data Store Read/1 -> Vxx_fms_phi_max_pinj2/1

== system AEMS_Standard_Library/SPECIFIC/AEMS_SUPPLIER_CALL_PHI_MAX_PINJ3 ==
  Data Store Read : DataStoreRead  DataStoreName=Supplier_Call_Phi_Max
      settings: AttributesFormatString=<tsample=%<sampleTime>>
  Vxx_fms_phi_max_pinj3 : Outport
  wires:
  Data Store Read/1 -> Vxx_fms_phi_max_pinj3/1

== system AEMS_Standard_Library/SPECIFIC/AEMS_SUPPLIER_CALL_PHI_MAX_PINJ4 ==
  Data Store Read : DataStoreRead  DataStoreName=Supplier_Call_Phi_Max
      settings: AttributesFormatString=<tsample=%<sampleTime>>
  Vxx_fms_phi_max_pinj4 : Outport
  wires:
  Data Store Read/1 -> Vxx_fms_phi_max_pinj4/1

== system AEMS_Standard_Library/SPECIFIC/AEMS_SUPPLIER_CALL_PHI_MIN_AFTR ==
  Data Store Read : DataStoreRead  DataStoreName=Supplier_Call_Phi_Min
      settings: AttributesFormatString=<tsample=%<sampleTime>>
  Vxx_fms_phi_min_aftr : Outport
  wires:
  Data Store Read/1 -> Vxx_fms_phi_min_aftr/1

== system AEMS_Standard_Library/SPECIFIC/AEMS_SUPPLIER_CALL_PHI_MIN_ING ==
  note: Coding information: This block is to call Supplier call API.
      | Each block will be translated into code C by this way:
      | Output=Supplier call API Name;
      | Example for Supplier_Call_Phi_min_post3, corresponding output variable is
      | Vxx_fms_phi_min_post3= Supplier_Call_Phi_min_post3;
  DataTypeConversion : DataTypeConversion
  Data_Store_Read : DataStoreRead  DataStoreName=Supplier_Call_Phi_min_post3
      settings: AttributesFormatString=<tsample=%<sampleTime>
  Vxx_fms_phi_min_post3 : Outport  InitialOutput=0
  wires:
  DataTypeConversion/1 -> Vxx_fms_phi_min_post3/1
  Data_Store_Read/1 -> DataTypeConversion/1

== system AEMS_Standard_Library/SPECIFIC/AEMS_SUPPLIER_CALL_PHI_MIN_LPOS ==
  Data Store Read : DataStoreRead  DataStoreName=Supplier_Call_Phi_Min
      settings: AttributesFormatString=<tsample=%<sampleTime>>
  Vxx_fms_phi_min_lpos1 : Outport
  wires:
  Data Store Read/1 -> Vxx_fms_phi_min_lpos1/1

== system AEMS_Standard_Library/SPECIFIC/AEMS_SUPPLIER_CALL_PHI_MIN_LPOS2 ==
  Data Store Read : DataStoreRead  DataStoreName=Supplier_Call_Phi_Min
      settings: AttributesFormatString=<tsample=%<sampleTime>>
  Vxx_fms_phi_min_lpos2 : Outport
  wires:
  Data Store Read/1 -> Vxx_fms_phi_min_lpos2/1

== system AEMS_Standard_Library/SPECIFIC/AEMS_SUPPLIER_CALL_PHI_MIN_LPOS3 ==
  Data Store Read : DataStoreRead  DataStoreName=Supplier_Call_Phi_Min
      settings: AttributesFormatString=<tsample=%<sampleTime>>
  Vxx_fms_phi_min_lpos3 : Outport
  wires:
  Data Store Read/1 -> Vxx_fms_phi_min_lpos3/1

== system AEMS_Standard_Library/SPECIFIC/AEMS_SUPPLIER_CALL_PHI_MIN_LPOS4 ==
  Data Store Read : DataStoreRead  DataStoreName=Supplier_Call_Phi_Min
      settings: AttributesFormatString=<tsample=%<sampleTime>>
  Vxx_fms_phi_min_lpos4 : Outport
  wires:
  Data Store Read/1 -> Vxx_fms_phi_min_lpos4/1
